simulink model "w2_prob4_214869"  (R2020a)
settings: Solver=VariableStepAuto  StartTime=0.0  StopTime=10.0  RelTol=1e-3
values from neighbouring files (symbols this model uses):
  B = 3.5077E-6    [w2_q4_214869.sldd]
  J = 3.2284E-6    [w2_q4_214869.sldd]
  K = 0.0274    [w2_q4_214869.sldd]
  L = 2.75E-6    [w2_q4_214869.sldd]
  R = 4.0    [w2_q4_214869.sldd]
settings Model: DataDictionary=w2_q4_214869.sldd  Creator=sonal  LastModifiedBy=sonal

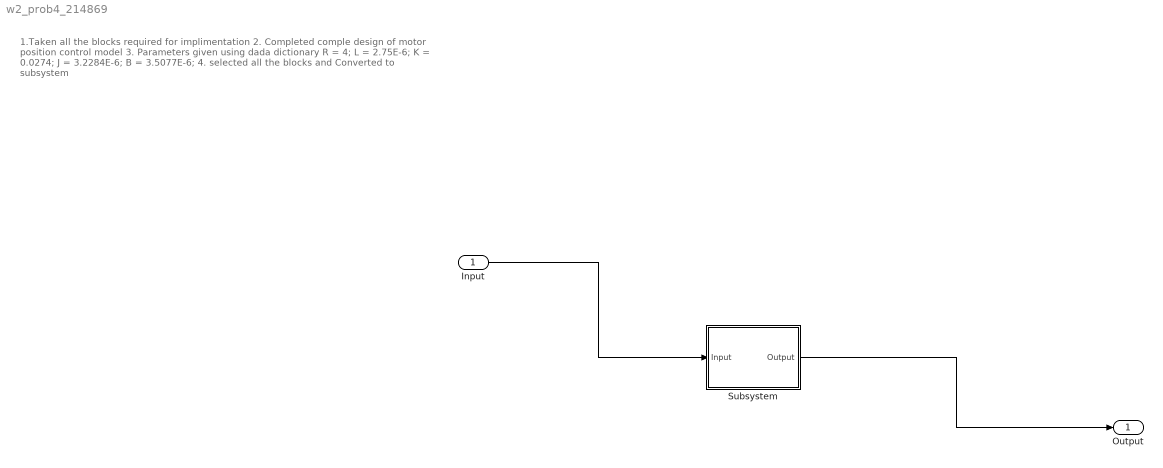
== system w2_prob4_214869 ==
  note: 1.Taken all the blocks required for implimentation
      |
      | 2. Completed comple design of motor position control model
      |
      | 3. Parameters given using dada dictionary
      | R = 4;
      | L = 2.75E-6;
      | K = 0.0274;
      | J = 3.2284E-6;
      | B = 3.5077E-6;
      | 4. selected all the blocks and Converted to subsystem
  Input : Inport
  Subsystem : Subsystem
  Output : Outport
  wires:
  Input/1 -> Subsystem/1(Input)
  Subsystem/1(Output) -> Output/1

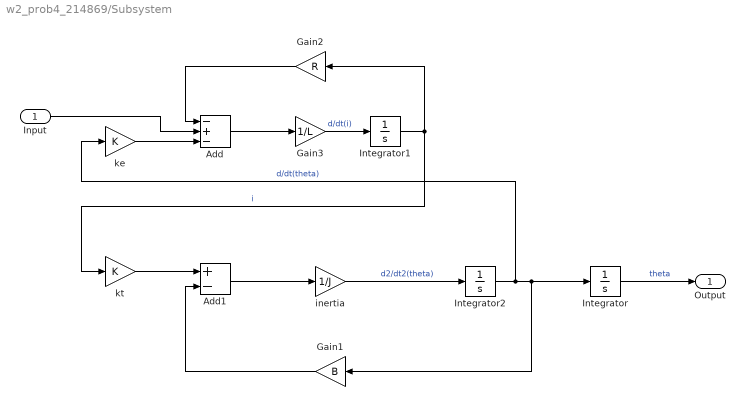
== system w2_prob4_214869/Subsystem ==
  Input : Inport
  Add : Sum  Inputs=-+-
  Add1 : Sum  Inputs=+-
  Gain1 : Gain  Gain=B
  Gain2 : Gain  Gain=R
  Gain3 : Gain  Gain=1/L
  Integrator : Integrator
  Integrator1 : Integrator
  Integrator2 : Integrator
  inertia : Gain  Gain=1/J
  ke : Gain  Gain=K
  kt : Gain  Gain=K
  Output : Outport
  wires:
  Gain2/1 -> Add/1
  Integrator2/1 -> ke/1, Gain1/1, Integrator/1  "d/dt(theta)"
  kt/1 -> Add1/1
  Gain3/1 -> Integrator1/1  "d/dt(i)"
  Add/1 -> Gain3/1
  ke/1 -> Add/3
  Input/1 -> Add/2
  Integrator/1 -> Output/1  "theta"
  Gain1/1 -> Add1/2
  Integrator1/1 -> Gain2/1, kt/1  "i"
  inertia/1 -> Integrator2/1  "d2/dt2(theta)"
  Add1/1 -> inertia/1
